simulink model "chap7_11sim"  (Simulink 5.0)
settings: Solver=ode45  StartTime=0.0  StopTime=20.0  FixedStep=0.001
settings Model: LastModifiedBy=Administrator  AlgebraicLoopMsg=none

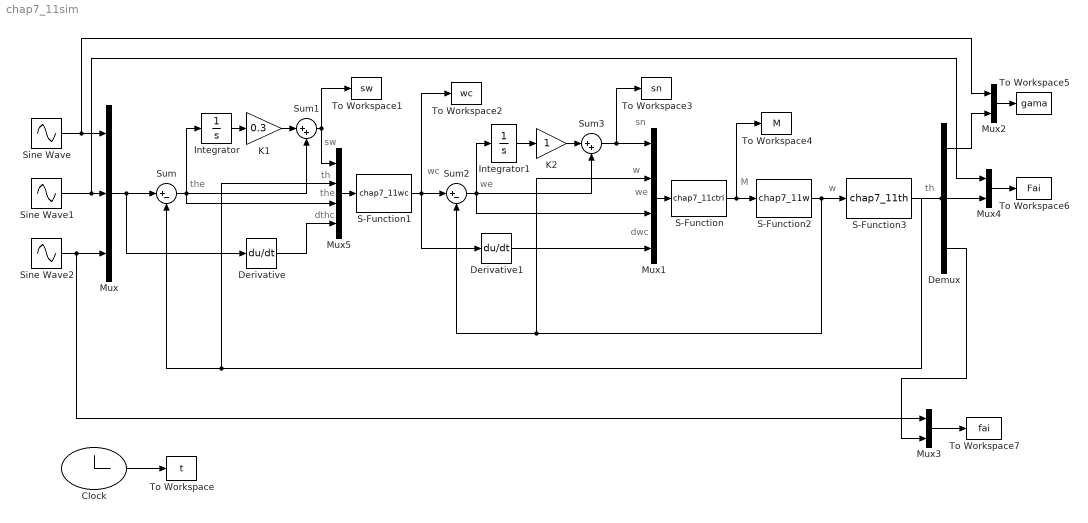
== system chap7_11sim ==
  note: sw
  note: th
  note: the
  note: dthc
  note: wc
  note: th
  note: w
  note: the
  note: we
  note: sn
  note: w
  note: we
  note: dwc
  note: M
  Clock : Clock
  Demux : Demux  Outputs=3
  Derivative : Derivative
  Derivative1 : Derivative
  Integrator : Integrator
  Integrator1 : Integrator
  K1 : Gain  Gain=0.3  SaturateOnIntegerOverflow=on
  K2 : Gain  SaturateOnIntegerOverflow=on
  Mux : Mux  Inputs=3
  Mux1 : Mux
  Mux2 : Mux  Inputs=2
  Mux3 : Mux  Inputs=2
  Mux4 : Mux  Inputs=2
  Mux5 : Mux
  S-Function : S-Function  FunctionName=chap7_11ctrl
  S-Function1 : S-Function  FunctionName=chap7_11wc
  S-Function2 : S-Function  FunctionName=chap7_11w
  S-Function3 : S-Function  FunctionName=chap7_11th
  Sine Wave : Sin  Phase=pi/2  SampleTime=0
  Sine Wave1 : Sin  Phase=pi/2  SampleTime=0
  Sine Wave2 : Sin  Phase=pi/2  SampleTime=0
  Sum : Sum  Inputs=|+-  SaturateOnIntegerOverflow=on
  Sum1 : Sum  Inputs=|++  SaturateOnIntegerOverflow=on
  Sum2 : Sum  Inputs=|+-  SaturateOnIntegerOverflow=on
  Sum3 : Sum  Inputs=|++  SaturateOnIntegerOverflow=on  InputSameDT=on
  To Workspace : ToWorkspace  VariableName=t  SampleTime=-1  SaveFormat=Array
  To Workspace1 : ToWorkspace  VariableName=sw  SampleTime=-1  SaveFormat=Array
  To Workspace2 : ToWorkspace  VariableName=wc  SampleTime=-1  SaveFormat=Array
  To Workspace3 : ToWorkspace  VariableName=sn  SampleTime=-1  SaveFormat=Array
  To Workspace4 : ToWorkspace  VariableName=M  SampleTime=-1  SaveFormat=Array
  To Workspace5 : ToWorkspace  VariableName=gama  SampleTime=-1  SaveFormat=Array
  To Workspace6 : ToWorkspace  VariableName=Fai  SampleTime=-1  SaveFormat=Array
  To Workspace7 : ToWorkspace  VariableName=fai  SampleTime=-1  SaveFormat=Array
  wires:
  Mux1/1 -> S-Function/1
  S-Function/1 -> S-Function2/1, To Workspace4/1
  S-Function2/1 -> Sum2/2, Mux1/2, S-Function3/1
  Sine Wave/1 -> Mux/1, Mux2/1
  S-Function3/1 -> Sum/2, Mux5/2, Demux/1
  Sum/1 -> Integrator/1, Mux5/3, Sum1/2
  Integrator/1 -> K1/1
  K1/1 -> Sum1/1
  Sum1/1 -> Mux5/1, To Workspace1/1
  Derivative/1 -> Mux5/4
  Mux5/1 -> S-Function1/1
  S-Function1/1 -> Sum2/1, Derivative1/1, To Workspace2/1
  Sum2/1 -> Mux1/3, Integrator1/1, Sum3/2
  Integrator1/1 -> K2/1
  K2/1 -> Sum3/1
  Sum3/1 -> Mux1/1, To Workspace3/1
  Derivative1/1 -> Mux1/4
  Mux/1 -> Sum/1, Derivative/1
  Sine Wave1/1 -> Mux/2, Mux4/1
  Sine Wave2/1 -> Mux/3, Mux3/1
  Demux/1 -> Mux2/2
  Mux2/1 -> To Workspace5/1
  Mux3/1 -> To Workspace7/1
  Demux/3 -> Mux3/2
  Mux4/1 -> To Workspace6/1
  Demux/2 -> Mux4/2
  Clock/1 -> To Workspace/1
